simulink model "Quattrini_Michael_0001070264"  (R2023b)
settings: Solver=FixedStepAuto  StartTime=0.0  StopTime=1.2  FixedStep=5.0e-7  RelTol=1e-3
values from neighbouring files (symbols this model uses):
  carrier_period = 1/carrier_frequency    (= 2.5e-06)    [Quattrini_Michael_p0001070264.m]
  current_saturation = 9.2    [Quattrini_Michael_p0001070264.m]
  kfi = 1/317 * (60/(2*pi))    (= 0.0301239639922)    [Quattrini_Michael_p0001070264.m]
  ki_c = 3050    [Quattrini_Michael_p0001070264.m]
  ki_w = 0.0001    [Quattrini_Michael_p0001070264.m]
  kp_c = 18    [Quattrini_Michael_p0001070264.m]
  kp_w = 0.150    (= 0.15)    [Quattrini_Michael_p0001070264.m]
  load_torque_slope = 5.856e-5    (= 5.856e-05)    [Quattrini_Michael_p0001070264.m]
  nominal_speed = 6930*2*pi/60    (= 725.707902979)    [Quattrini_Michael_p0001070264.m]
  source_internal_resistance = 0.30    (= 0.3)    [Quattrini_Michael_p0001070264.m]
  supply_voltage = 30    [Quattrini_Michael_p0001070264.m]
  total_inertia = (rotor_inertia + load_inertia) * 10^(-7)    (= 3.38e-05)    [Quattrini_Michael_p0001070264.m]
  winding_resistance = 0.32    [Quattrini_Michael_p0001070264.m]
libraries: nesl_utility x12, ee_lib x10, fl_lib x8, simulink x3
settings Model: Creator=vince  LastModifiedBy=Utente
settings ModelReferenceCC: EnableRefExpFcnMdlSchedulingChecks=on

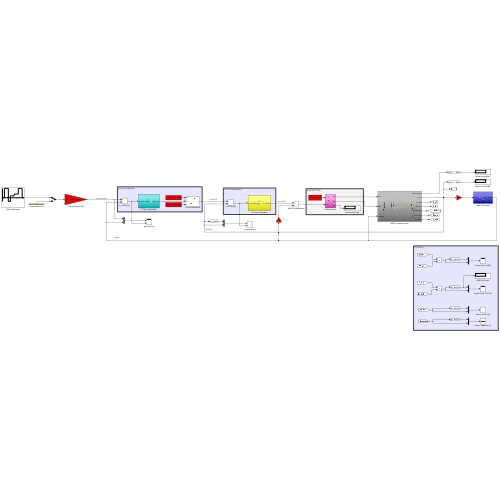
[thumbnail: Simulink's stored preview of the top-level diagram]
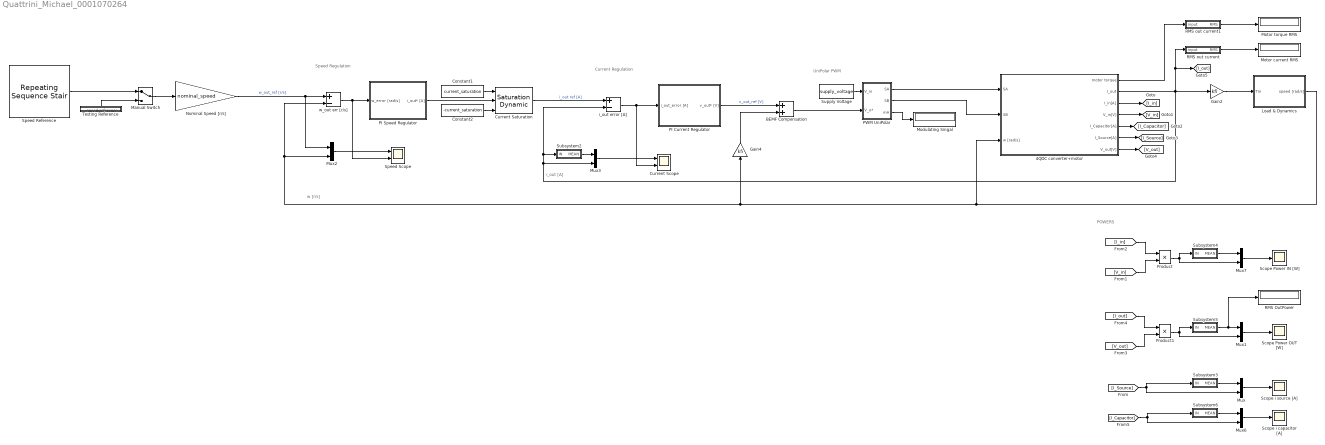
== system Quattrini_Michael_0001070264 ==
  note: w [r/s]
  note: i_out [A]
  note: Speed Regulation
  note: Current Regulation
  note: UniPolar PWM
  note: POWERS
  4QDC converter+motor : Subsystem
  BEMF Compensation : Sum
  Constant1 : Constant  Value=current_saturation
  Constant2 : Constant  Value=-current_saturation
  Current Saturation : simulink/Discontinuities/Saturation Dynamic  OutMin=[]  OutMax=[]  OutDataTypeStr=Inherit: Same as second input  OutDataType=fixdt(1, 16)  OutScaling=2^-10  DoSatur=off
  Current Scope : Scope  NumInputPorts=2
  Gain2 : Gain  Gain=kfi
  Gain4 : Gain  Gain=kfi
  Load & Dynamics : Subsystem
  Manual Switch : ManualSwitch
  Modulating Singal : Display
  Motor current RMS : Display
  Motor torque RMS : Display
  Mux{,1..3,6..7} (6 alike) : Mux  Inputs=2
  Nominal Speed [r/s] : Gain  Gain=nominal_speed
  PI Current Regulator : Subsystem
  PI Speed Regulator : Subsystem
  PWM UniPolar : Subsystem
  Product : Product
  Product1 : Product
  RMS OutPower : Display
  RMS out current : Subsystem  mask{t=1.2}
      mask prompts: t "Integrating time T [s]"
      mask DialogControl DescTextVar Prompt: Mean value calculator over period T
  RMS out current1 : Subsystem  mask{t=1.2}
      mask prompts: t "Integrating time T [s]"
      mask DialogControl DescTextVar Prompt: Mean value calculator over period T
  Scope Power IN [W] : Scope
  Scope Power OUT [W] : Scope
  Scope i capacitor [A] : Scope
  Scope i source [A] : Scope
  Speed Reference : simulink/Sources/Repeating Sequence Stair  OutValues=[0 1.25 1.25 -0.5 0.25 0.25 0.50 0.50 1.25 1.25 1/667^2]  tsamp=0.1  OutMin=[]  OutMax=[]  OutDataTypeStr=double  OutputDataTypeScalingMode=double  OutDataType=fixdt(0,8)  ConRadixGroup=Best Precision: Vector-wise  OutScaling=2^-12
  Speed Scope : Scope  NumInputPorts=2
  Subsystem2 : Subsystem  mask{carrierPeriod=carrier_period}
  Subsystem3 : Subsystem  mask{carrierPeriod=carrier_period}
  Subsystem4 : Subsystem  mask{carrierPeriod=carrier_period}
  Subsystem5 : Subsystem  mask{carrierPeriod=carrier_period}
  Subsystem6 : Subsystem  mask{carrierPeriod=carrier_period}
  Supply Voltage : Constant  Value=supply_voltage
  Testing Reference : Subsystem
      settings: PortSchema="{\"entries\":[{\"content\":{\"sides\":[{\"content\":{\"connectorIds\":[]},\"type\":\"ConnectorPlacement.EquallySpacedRectSide\",\"uuid\":\"1e7059c8-be33-4535-aff5-f50a3743a179\"},{\"content\":{\"connectorIds\":[],\"side\":\"RIGHT\"},\"type\":\"ConnectorPlacement.EquallySpacedRectSide\",\"uuid\":\"f13681df-83b1-4c0d-b4d9-acb75cd15713\"},{\"content\":{\"connectorIds\":[\"Out1\"],\"side\":\"TOP\"},\"type\":\"ConnectorPlacement.EquallySpacedRectSide\",\"uuid\":\"954c28a6-7a50-41b4-bd4f-7c1c0b7465e3\"}]},\"type\":\"ConnectorPlacement.EquallySpacedConnector\",\"uuid\":\"8215162a-5d8c-4681-a7f6-9e1221fb7294\"}],\"packageUris\":[\"http://schema.mathworks.com/mf0/Connector/R2020b\"],\"version\":\"1.0\"}"
  i_out error [A] : Sum  Inputs=+-
  w_out err [r/s] : Sum  Inputs=+-
  wires:
  BEMF Compensation/1 -> PWM UniPolar/2(V_o*)
  Current Saturation/1 -> i_out error [A]/1  "i_out ref [A]"
  i_out error [A]/1 -> PI Current Regulator/1(i_out_error [A]), Current Scope/2
  w_out err [r/s]/1 -> Speed Scope/2, PI Speed Regulator/1(w_error [rad/s])
  Nominal Speed [r/s]/1 -> w_out err [r/s]/1, Mux2/1  "w_out_ref [r/s]"
  Gain4/1 -> BEMF Compensation/2
  Subsystem2/1(MEAN) -> Mux3/1
  PI Speed Regulator/1(i_out* [A]) -> Current Saturation/2
  Constant1/1 -> Current Saturation/1
  Manual Switch/1 -> Nominal Speed [r/s]/1
  Speed Reference/1 -> Manual Switch/1
  Testing Reference/1(speed reference) -> Manual Switch/2
  Gain2/1 -> Load & Dynamics/1(Tm)
  Load & Dynamics/1(speed [rad/s]) -> Gain4/1, w_out err [r/s]/2, Mux2/2, 4QDC converter+motor/3(w [rad/s])
  Supply Voltage/1 -> PWM UniPolar/1(V_in)
  PWM UniPolar/3(mA) -> Modulating Singal/1
  PWM UniPolar/2(SB) -> 4QDC converter+motor/2(SB)
  PWM UniPolar/1(SA) -> 4QDC converter+motor/1(SA)
  Mux3/1 -> Current Scope/1
  Mux2/1 -> Speed Scope/1
  PI Current Regulator/1(v_out* [V]) -> BEMF Compensation/1  "v_out_ref [V]"
  4QDC converter+motor/2(I_out) -> Mux3/2, Subsystem2/1(IN), i_out error [A]/2, Gain2/1, RMS out current/1(input), [I_out]
  4QDC converter+motor/3(I_in[A]) -> [I_in]
  4QDC converter+motor/4(V_in[V]) -> [V_in]
  4QDC converter+motor/6(I_Source[A]) -> [I_Source]
  4QDC converter+motor/5(I_Capacitor[A]) -> [I_Capacitor]
  RMS out current1/1(RMS) -> Motor torque RMS/1
  RMS out current/1(RMS) -> Motor current RMS/1
  4QDC converter+motor/1(motor torque) -> RMS out current1/1(input)
  Product/1 -> Mux7/2, Subsystem4/1(IN)
  Subsystem4/1(MEAN) -> Mux7/1
  [V_out] -> Product1/2
  [V_in] -> Product/2
  [I_out] -> Product1/1
  Product1/1 -> Mux1/2, Subsystem5/1(IN)
  Mux1/1 -> Scope Power OUT [W]/1
  Subsystem5/1(MEAN) -> RMS OutPower/1, Mux1/1
  [I_in] -> Product/1
  Mux7/1 -> Scope Power IN [W]/1
  [I_Source] -> Subsystem3/1(IN), Mux/2
  Mux6/1 -> Scope i capacitor [A]/1
  Subsystem3/1(MEAN) -> Mux/1
  Mux/1 -> Scope i source [A]/1
  [I_Capacitor] -> Mux6/2, Subsystem6/1(IN)
  Subsystem6/1(MEAN) -> Mux6/1
  Constant2/1 -> Current Saturation/3
  4QDC converter+motor/7(V_out[V]) -> [V_out]

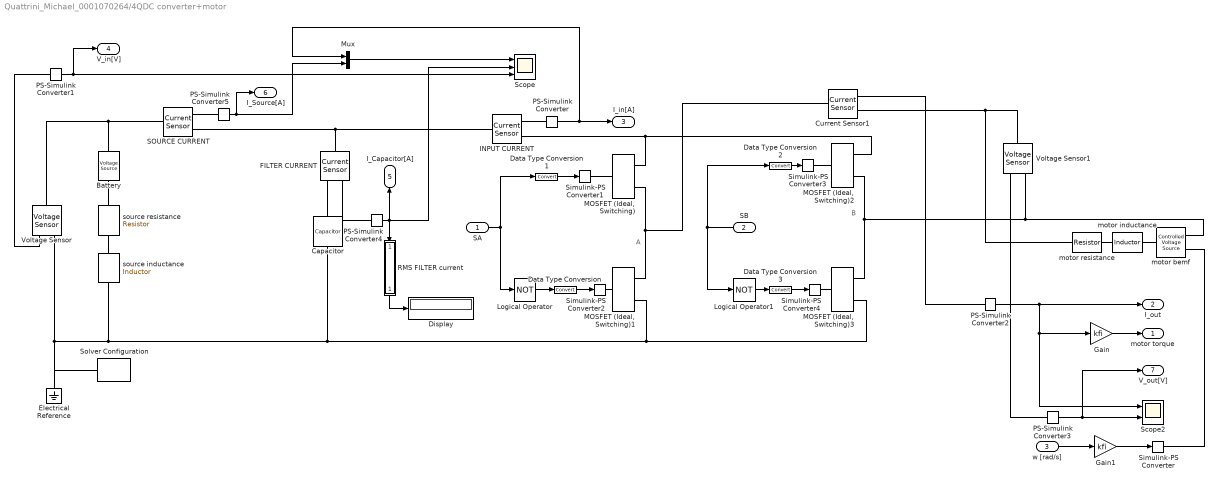
== system Quattrini_Michael_0001070264/4QDC converter+motor ==
  note: B
  note: A
  SA : Inport
  SB : Inport  Port=2
  w [rad/s] : Inport  Port=3
  Battery : ee_lib/Sources/Voltage Source  dc_voltage=supply_voltage V  ac_voltage=0 V  ac_shift=0 rad  ac_frequency=60 Hz  noise_mode=0  PSD=0 V^2/Hz  sample_time=1e-3 s  repeatability=1  user_seed=0  auto_seed=3890346746  i_specify=off  i_priority=None  i=0 A  i_nominal_specify=off  i_nominal_unit=A  i_nominal_value=1  v_specify=off  v_priority=None  v=0 V  v_nominal_specify=off  v_nominal_unit=V  v_nominal_value=1
  Capacitor : ee_lib/Passive/Capacitor  cap_option=ee.enum.passive.capacitor.capOption.const  c=filter_capacitance F  Cvec=[1e-05, 1e-06] F  Vvec=[0, 10] V  CV_table_symmetry=1  f_vec=[1, 10] kHz  DFext_vec=[.8, 1.2]  enable_C_tol=0  averaging_period=0 s  C_tol=5  tol_distribution=1  nSigma=4  r=0.001 Ohm  g=0 1/Ohm  enable_operating_limits=0  operating_limit_action=2  max_working_voltage_range=[-25, 25] V  power_rating=1 W  enable_faults=ee.enum.enable.no  fault_action=simscape.enum.assert.action.none  Cscale_faulted=100  R_faulted=1e-3 Ohm  G_faulted=0 1/Ohm  tau_fault=1e-3 s  fault_trigger=ee.enum.faults.faultTrigger.temporal  t_fault=1 s  max_permissible_voltage_range=[-100, 100] V  t_fail_on_voltage=1 s  i_specify=off  i_priority=None  i=0 A  i_nominal_specify=off  i_nominal_unit=A  i_nominal_value=1  v_specify=off  v_priority=None  v=0 V  v_nominal_specify=off  v_nominal_unit=V  v_nominal_value=1  vc_specify=off  vc_priority=High  vc=0 V  vc_nominal_specify=off  vc_nominal_unit=V  vc_nominal_value=1
  Current Sensor1 : fl_lib/Electrical/Electrical Sensors/Current Sensor
  Data Type Conversion{,1..3} (4 alike) : DataTypeConversion  SaturateOnIntegerOverflow=off  RndMeth=Floor
  Display : Display
  Electrical Reference : fl_lib/Electrical/Electrical Elements/Electrical Reference
  FILTER CURRENT : fl_lib/Electrical/Electrical Sensors/Current Sensor
  Gain : Gain  Gain=kfi
  Gain1 : Gain  Gain=kfi
  INPUT CURRENT : fl_lib/Electrical/Electrical Sensors/Current Sensor
  Logical Operator : Logic  Operator=NOT  AllPortsSameDT=off  OutDataTypeStr=boolean
  Logical Operator1 : Logic  Operator=NOT  AllPortsSameDT=off  OutDataTypeStr=boolean
  MOSFET (Ideal, Switching){,1..3} (4 alike) : ee_lib/Semiconductors & Converters/MOSFET (Ideal, Switching)  port_option=ee.enum.controlport.ps  Rds=0.01 Ohm  Goff=1e-6 1/Ohm  Vth=0.5 V  diode_param=1  diode_Vf=0.8 V  diode_Ron=0.001 Ohm  diode_Goff=1e-5 1/Ohm  diode_C=50e-9 F  diode_iRM=-235 A  diode_iF=300 A  diode_idot=-50 A/us  diode_trr_param=1  diode_trr_factor=3  diode_trr=15 us  diode_Qrr=1500 s*uA  ids_specify=off  ids_priority=None  ids=0 A  ids_nominal_specify=off  ids_nominal_unit=A  ids_nominal_value=1  vds_specify=off  vds_priority=None  vds=0 V  vds_nominal_specify=off  vds_nominal_unit=V  vds_nominal_value=1  vgs_specify=off  vgs_priority=None  vgs=0 V  vgs_nominal_specify=off  vgs_nominal_unit=V  vgs_nominal_value=1  thermal_loss_option=ee.enum.converters.thermalLossOption.constantvalues  Von_data=[0, 1.8, 3.2, 6, 10, 16; 0, 2, 5.5, 9.5, 15, 25] V  Tj=[298.15, 448.15] K  Iout_data=[0, 20, 40, 60, 80, 100] A  Eon_data=[0, 55.04, 124.57, 235.53, 362.12; 0, 71.25, 161.25, 304.88, 468.75] * 1e-6 J  Eoff_data=[0, 18, 30, 56.1, 76.5; 0, 22.5, 37.5, 70.13, 95.63] * 1e-6 J  Eon_data_3D=[zeros(2, 5, 3)] J  Eoff_data_3D=[zeros(2, 5, 3)] J  Tj_loss=[298.15, 448.15] K  Iout_data_loss=[0, 10, 20, 30, 40] A  tabulateWithVds=false  Vds_loss=[0, 150, 300] V  Eon_scalar=22.86e-3 J  Eoff_scalar=17.14e-3 J  Voff=300 V  Iout_scalar=600 A  useCurrentFromPreviousCycle=false  useVoltageFromPreviousCycle=false  diodeModelType=ee.enum.converters.diodeModelType.pwl  diodeTableType=ee.enum.diode.tableType.IfMat  diode_IfMat=[.07, .12, .19, 1.75, 4.24, 7.32, 11.2; .16, .3, .72, 2.14, 4.02, 6.35, 9.12] A  diode_VfMat=[.9, 1.15, 1.25, 1.5, 1.75, 2.17, 2.6, 2.85; .58, .68, .75, 1.1, 1.38, 1.77, 2.27, 2.7] V  diode_TjVec=[25, 125] degC  diode_VfVec=[.5, .7, .9, 1.3, 1.7, 2.1, 2.5] V  diode_IfVec=[.1, .2, .5, 1, 2, 4, 7, 10] A  diode_Vr=-600 V  diode_Ls=150 nH  diode_Erec=0.03 J  diode_rec_loss_model=ee.enum.diode.reverseRecoveryModel.fixed  diode_ErecVal=0 J  diode_scaleWithIandV=true  diode_ErecMat=zeros(2, 3) J  diode_TjrecVec=[298.15, 398.15] K  diode_IfrecVec=[.1, 1, 10] A  diode_IrecVal=10 A  diode_VrecVal=10 V  diode_tFilter=1 / 1000 / 100 s  thermal_network_parameterization=ee.enum.thermalNetworkTopology.external  Rth=[.03, .2] K/W  Rth_Cauer=[.03, .1, .2] K/W  Rth_Foster=[.03, .2] K/W  thermal_mass_parameterization=ee.enum.thermalNetwork.timeconstant  thermal_mass=[3, 25] J/K  thermal_mass_Cauer=[3, 10, 25] J/K  thermal_mass_Foster=[33, 50] J/K  thermal_time_constant=[.1, 5] s  thermal_time_constant_Cauer=[.1, 1, 5] s  thermal_time_constant_Foster=[1, 10] s  thermal_mass_initial_temperatures=[25, 25] degC  thermal_mass_initial_temperatures_Cauer=[25, 25, 25] degC  junction_thermal_mass=0.1 J/K  Tvec_initial_Foster=[25, 25, 25, 25] degC  no_thermal_network=0  junction_temperature_specify=off  junction_temperature_priority=None  junction_temperature=25 degC  junction_temperature_nominal_specify=off  junction_temperature_nominal_unit=degC  junction_temperature_nominal_value=1  Qj_specify=off  Qj_priority=None  Qj=0 W  Qj_nominal_specify=off  Qj_nominal_unit=W  Qj_nominal_value=1  accumulatedSwitchingLosses_specify=off  accumulatedSwitchingLosses_priority=None  accumulatedSwitchingLosses=0 J
  Mux : Mux  Inputs=2
  PS-Simulink Converter{,1..5} (6 alike) : nesl_utility/PS-Simulink Converter  PhysicalDomain=network_engine_domain  SubClassName=ps_output  LeftPortType=input  RightPortType=output  PseudoPeriodic=off  Frequencies=[]  VectorFormat=1-D array  Unit=inherit  AffineConversion=off
  RMS FILTER current : Subsystem  mask{t=1.2}
      mask prompts: t "Integrating time T [s]"
      mask DialogControl DescTextVar Prompt: Mean value calculator over period T
  SOURCE CURRENT : fl_lib/Electrical/Electrical Sensors/Current Sensor
  Scope : Scope  NumInputPorts=3
  Scope2 : Scope  NumInputPorts=2
  Simulink-PS Converter{,1..4} (5 alike) : nesl_utility/Simulink-PS Converter  PhysicalDomain=network_engine_domain  SubClassName=ps_input  LeftPortType=input  RightPortType=output  PseudoPeriodic=off  Frequencies=[]  NoiseDistribution=none  NoiseParameters=[]  Unit=1  AffineConversion=off  FilteringAndDerivatives=provide  SimscapeFilterOrder=1  InputFilterTimeConstant=0.001  UdotUserProvided=0
  Solver Configuration : nesl_utility/Solver Configuration  PhysicalDomain=network_engine_domain  SubClassName=solver  LeftPortType=input  RightPortType=generic  Tones=[]  Harmonics=[]  SimulateNoise=off  Profile=off  UseLocalSampling=off  EnableSwitchedLinearOptims=on  FrequencyDomain=off  UseCCode=off  RelTol=0.001  AbsTol=1e-06  MinStep=1e-09  ToWorkspace=off  RevertToSquareIcSolve=off  NumHomotopyIterations=100  PhasorMode=off  PhasorModeNumHarmonics=1  ConsistencySolver=NEWTON_FTOL  IndexReductionMethod=DerivativeReplacement  DoDC=off  ResidualTolerance=1e-09  ConsistencyTolSource=GLOBAL  ConsistencyAbsTol=0.001  ConsistencyRelTol=0.001  ConsistencyTolFactor=0.001  UseLocalSolver=off  LocalSolverChoice=NE_BACKWARD_EULER_ADVANCER  ResolveIndetEquations=on  FunctionEvalNumThread=1  LocalSolverSampleTime=0.001  DoFixedCost=off  MaxNonlinIter=3  MaxModeIter=2  ComputeImpulses=off  ImpulseIterations=2  LinearAlgebra=auto  LinearAlgebraNumThread=0  EquationFormulation=NE_TIME_EF  DelaysMemoryBudget=1024  AutomaticFiltering=on  FilteringTimeConstant=0.001  PartitionStorageMethod=AS_NEEDED  PartitionMemoryBudget=1024  PartitionMethod=ROBUST  MultibodyUseLocalSolver=off  MultibodyLocalSolverChoice=ODE1  MultibodyLocalSolverSampleTime=0.001
  Voltage Sensor : fl_lib/Electrical/Electrical Sensors/Voltage Sensor
  Voltage Sensor1 : fl_lib/Electrical/Electrical Sensors/Voltage Sensor
  motor inductance : ee_lib/Passive/Inductor  l=winding_inductance H  enable_L_tol=0  L_tol=20  tol_distribution=1  nSigma=4  r=0 Ohm  g=1e-9 1/Ohm  enable_operating_limits=0  operating_limit_action=2  max_working_current=1 A  power_rating=1 W  enable_faults=ee.enum.enable.no  fault_action=simscape.enum.assert.action.none  lambdaPercent=50  k_faulted=0.9999  turnsShort=0  openCct=0  groundShort=0  groundShortG=0 1/Ohm  tau_fault=1e-3 s  fault_trigger=ee.enum.faults.faultTrigger.temporal  t_fault=1 s  max_permissible_voltage=100 V  n_fail_on_voltage=1  max_permissible_current=1 A  t_fail_on_current=1 s  i_L_specify=off  i_L_priority=High  i_L=0 A  i_L_nominal_specify=off  i_L_nominal_unit=A  i_L_nominal_value=1
  "motor resistance " : ee_lib/Passive/Resistor  R=winding_resistance Ohm  enable_R_tol=0  R_tol=5  tol_distribution=1  nSigma=4  enable_operating_limits=0  operating_limit_action=2  power_rating=1 W  max_working_voltage=100 V  enable_faults=ee.enum.enable.no  fault_action=simscape.enum.assert.action.none  R_faulted=inf Ohm  fault_trigger=ee.enum.faults.faultTrigger.temporal  t_fault=1 s  max_permissible_current=1 A  t_fail_on_current=1 s  noise_mode=0  Tdevice=25 degC  sample_time=1e-3 s  repeatability=1  user_seed=0  auto_seed=545404223  faulted_specify=off  faulted_priority=None  faulted=0  power_derating_T1=70 degC  power_derating_T2=155 degC  operating_temperature_range_vec=[-50, 150] degC  alpha=3.93e-3 1/K  Tmeas=25 degC  thermal_mass=100 J/K  temperature_specify=off  temperature_priority=High  temperature=298.15 K  temperature_nominal_specify=off  temperature_nominal_unit=K  temperature_nominal_value=1
  motor bemf : fl_lib/Electrical/Electrical Sources/Controlled Voltage Source
  source inductance : ee_lib/Passive/Inductor  l=source_internal_inductance H  enable_L_tol=0  L_tol=20  tol_distribution=1  nSigma=4  r=0 Ohm  g=1e-9 1/Ohm  enable_operating_limits=0  operating_limit_action=2  max_working_current=1 A  power_rating=1 W  enable_faults=ee.enum.enable.no  fault_action=simscape.enum.assert.action.none  lambdaPercent=50  k_faulted=0.9999  turnsShort=0  openCct=0  groundShort=0  groundShortG=0 1/Ohm  tau_fault=1e-3 s  fault_trigger=ee.enum.faults.faultTrigger.temporal  t_fault=1 s  max_permissible_voltage=100 V  n_fail_on_voltage=1  max_permissible_current=1 A  t_fail_on_current=1 s  i_L_specify=off  i_L_priority=High  i_L=0 A  i_L_nominal_specify=off  i_L_nominal_unit=A  i_L_nominal_value=1
  source resistance : ee_lib/Passive/Resistor  R=source_internal_resistance Ohm  enable_R_tol=0  R_tol=5  tol_distribution=1  nSigma=4  enable_operating_limits=0  operating_limit_action=2  power_rating=1 W  max_working_voltage=100 V  enable_faults=ee.enum.enable.no  fault_action=simscape.enum.assert.action.none  R_faulted=inf Ohm  fault_trigger=ee.enum.faults.faultTrigger.temporal  t_fault=1 s  max_permissible_current=1 A  t_fail_on_current=1 s  noise_mode=0  Tdevice=25 degC  sample_time=1e-3 s  repeatability=1  user_seed=0  auto_seed=3922919431  faulted_specify=off  faulted_priority=None  faulted=0  power_derating_T1=70 degC  power_derating_T2=155 degC  operating_temperature_range_vec=[-50, 150] degC  alpha=3.93e-3 1/K  Tmeas=25 degC  thermal_mass=100 J/K  temperature_specify=off  temperature_priority=High  temperature=298.15 K  temperature_nominal_specify=off  temperature_nominal_unit=K  temperature_nominal_value=1
  motor torque : Outport
  I_out : Outport  Port=2
  I_in[A] : Outport  Port=3
  V_in[V] : Outport  Port=4
  I_Capacitor[A] : Outport  Port=5
  I_Source[A] : Outport  Port=6
  V_out[V] : Outport  Port=7
  wires:
  SB/1 -> Data Type Conversion2/1, Logical Operator1/1
  SA/1 -> Logical Operator/1, Data Type Conversion1/1
  PS-Simulink Converter2/1 -> Scope2/1, Gain/1, I_out/1
  Gain/1 -> motor torque/1
  w [rad/s]/1 -> Gain1/1
  Gain1/1 -> Simulink-PS Converter/1
  PS-Simulink Converter3/1 -> V_out[V]/1, Scope2/2
  Logical Operator/1 -> Data Type Conversion/1
  Data Type Conversion/1 -> Simulink-PS Converter2/1
  Data Type Conversion1/1 -> Simulink-PS Converter1/1
  Data Type Conversion2/1 -> Simulink-PS Converter3/1
  Logical Operator1/1 -> Data Type Conversion3/1
  Data Type Conversion3/1 -> Simulink-PS Converter4/1
  PS-Simulink Converter/1 -> Mux/1, I_in[A]/1
  Mux/1 -> Scope/1
  PS-Simulink Converter1/1 -> V_in[V]/1, Scope/3
  PS-Simulink Converter5/1 -> I_Source[A]/1, Mux/2
  PS-Simulink Converter4/1 -> I_Capacitor[A]/1, Scope/2, RMS FILTER current/1(input)
  RMS FILTER current/1(RMS) -> Display/1
  connections:
  Voltage Sensor/LConn1 -- Battery/LConn1 -- SOURCE CURRENT/LConn1
  "MOSFET (Ideal, Switching)1"/RConn2 -- Capacitor/RConn1 -- Voltage Sensor/RConn2 -- Electrical Reference/LConn1 -- Solver Configuration/RConn1 -- source inductance/RConn1 -- "MOSFET (Ideal, Switching)3"/RConn2
  "motor resistance "/RConn1 -- motor inductance/LConn1
  Simulink-PS Converter3/RConn1 -- "MOSFET (Ideal, Switching)2"/LConn1
  INPUT CURRENT/RConn2 -- "MOSFET (Ideal, Switching)"/RConn1 -- "MOSFET (Ideal, Switching)2"/RConn1
  motor bemf/RConn2 -- "MOSFET (Ideal, Switching)2"/RConn2 -- "MOSFET (Ideal, Switching)3"/RConn1 -- Voltage Sensor1/RConn2
  INPUT CURRENT/RConn1 -- PS-Simulink Converter/LConn1
  Voltage Sensor/RConn1 -- PS-Simulink Converter1/LConn1
  Simulink-PS Converter1/RConn1 -- "MOSFET (Ideal, Switching)"/LConn1
  Simulink-PS Converter/RConn1 -- motor bemf/RConn1
  "MOSFET (Ideal, Switching)"/RConn2 -- Current Sensor1/LConn1 -- "MOSFET (Ideal, Switching)1"/RConn1
  Simulink-PS Converter4/RConn1 -- "MOSFET (Ideal, Switching)3"/LConn1
  Simulink-PS Converter2/RConn1 -- "MOSFET (Ideal, Switching)1"/LConn1
  motor inductance/RConn1 -- motor bemf/LConn1
  Current Sensor1/RConn2 -- Voltage Sensor1/LConn1 -- "motor resistance "/LConn1
  Current Sensor1/RConn1 -- PS-Simulink Converter2/LConn1
  Voltage Sensor1/RConn1 -- PS-Simulink Converter3/LConn1
  source inductance/LConn1 -- source resistance/RConn1
  source resistance/LConn1 -- Battery/RConn1
  SOURCE CURRENT/RConn2 -- FILTER CURRENT/LConn1 -- INPUT CURRENT/LConn1
  FILTER CURRENT/RConn2 -- Capacitor/LConn1
  FILTER CURRENT/RConn1 -- PS-Simulink Converter4/LConn1
  SOURCE CURRENT/RConn1 -- PS-Simulink Converter5/LConn1

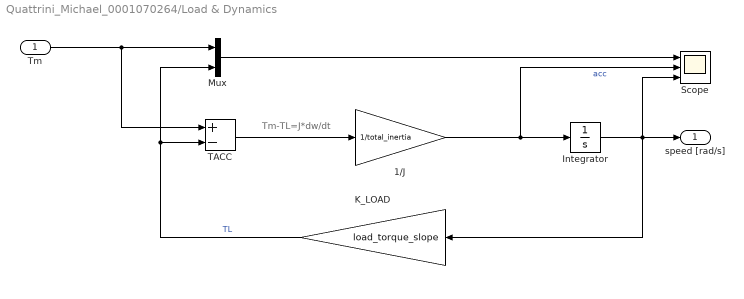
== system Quattrini_Michael_0001070264/Load & Dynamics ==
  note: Tm-TL=J*dw/dt
  Tm : Inport
  1/J : Gain  Gain=1/total_inertia
  Integrator : Integrator
  K_LOAD : Gain  Gain=load_torque_slope
  Mux : Mux  Inputs=2
  Scope : Scope  NumInputPorts=3
  TACC : Sum  Inputs=+-
  speed [rad/s] : Outport
  wires:
  Tm/1 -> Mux/1, TACC/1
  1/J/1 -> Scope/2, Integrator/1  "acc"
  K_LOAD/1 -> Mux/2, TACC/2  "TL"
  Integrator/1 -> K_LOAD/1, Scope/3, speed [rad/s]/1
  TACC/1 -> 1/J/1
  Mux/1 -> Scope/1

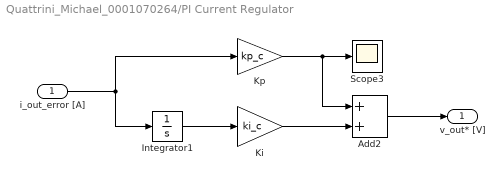
== system Quattrini_Michael_0001070264/PI Current Regulator ==
  i_out_error [A] : Inport
  Add2 : Sum
  Integrator1 : Integrator
  Ki : Gain  Gain=ki_c
  Kp : Gain  Gain=kp_c
  Scope3 : Scope
  v_out* [V] : Outport
  wires:
  Add2/1 -> v_out* [V]/1
  Kp/1 -> Add2/1, Scope3/1
  Ki/1 -> Add2/2
  Integrator1/1 -> Ki/1
  i_out_error [A]/1 -> Kp/1, Integrator1/1

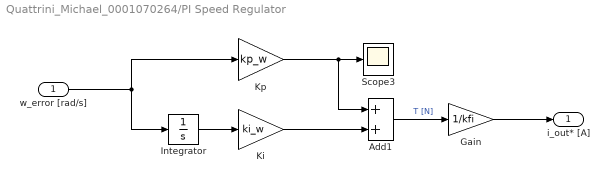
== system Quattrini_Michael_0001070264/PI Speed Regulator ==
  w_error [rad/s] : Inport
  Add1 : Sum
  Gain : Gain  Gain=1/kfi
  Integrator : Integrator
  Ki : Gain  Gain=ki_w
  Kp : Gain  Gain=kp_w
  Scope3 : Scope
  i_out* [A] : Outport
  wires:
  w_error [rad/s]/1 -> Integrator/1, Kp/1
  Kp/1 -> Add1/1, Scope3/1
  Integrator/1 -> Ki/1
  Ki/1 -> Add1/2
  Add1/1 -> Gain/1  "T [N]"
  Gain/1 -> i_out* [A]/1

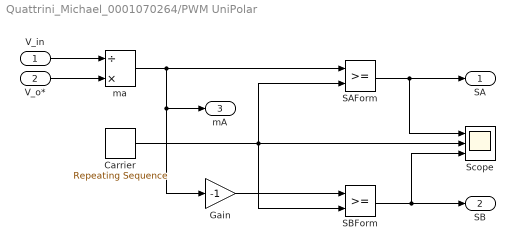
== system Quattrini_Michael_0001070264/PWM UniPolar ==
  V_in : Inport
  V_o* : Inport  Port=2
  Carrier : simulink/Sources/Repeating Sequence  rep_seq_t=[0 carrier_period/2 carrier_period]  rep_seq_y=[-1 1 -1]
  Gain : Gain  Gain=-1
  SAForm : RelationalOperator  OutDataTypeStr=boolean  RndMeth=Simplest  InputSameDT=off
  SBForm : RelationalOperator  OutDataTypeStr=boolean  RndMeth=Simplest  InputSameDT=off
  Scope : Scope  NumInputPorts=3
  ma : Product  Inputs=/*
  SA : Outport
  SB : Outport  Port=2
  mA : Outport  Port=3
  wires:
  Carrier/1 -> SBForm/2, SAForm/2, Scope/2
  Gain/1 -> SBForm/1
  SBForm/1 -> SB/1, Scope/3
  SAForm/1 -> Scope/1, SA/1
  V_in/1 -> ma/1
  V_o*/1 -> ma/2
  ma/1 -> mA/1, Gain/1, SAForm/1

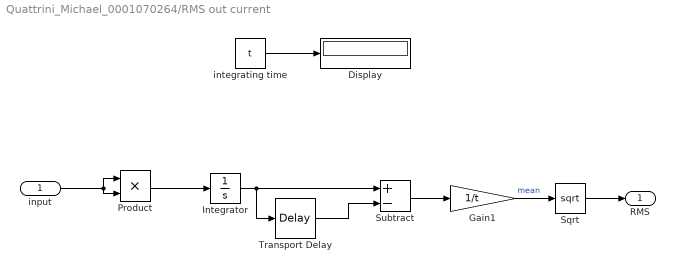
== system Quattrini_Michael_0001070264/RMS out current ==
  input : Inport
  Display : Display
  Gain1 : Gain  Gain=1/t
  Integrator : Integrator
  Product : Product
  Sqrt : Sqrt
  Subtract : Sum  Inputs=+-
  Transport Delay : TransportDelay  DelayTime=t
  integrating time : Constant  Value=t
  RMS : Outport
  wires:
  integrating time/1 -> Display/1
  Transport Delay/1 -> Subtract/2
  Integrator/1 -> Transport Delay/1, Subtract/1
  Subtract/1 -> Gain1/1
  input/1 -> Product/1, Product/2
  Product/1 -> Integrator/1
  Sqrt/1 -> RMS/1
  Gain1/1 -> Sqrt/1  "mean"

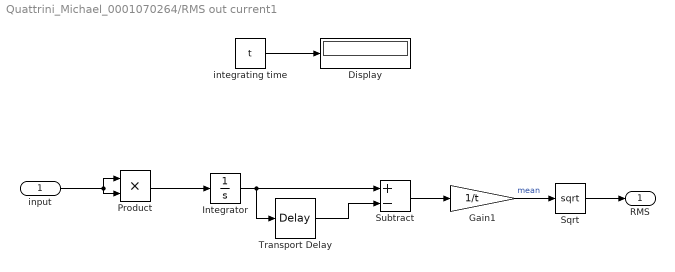
== system Quattrini_Michael_0001070264/RMS out current1 ==
  input : Inport
  Display : Display
  Gain1 : Gain  Gain=1/t
  Integrator : Integrator
  Product : Product
  Sqrt : Sqrt
  Subtract : Sum  Inputs=+-
  Transport Delay : TransportDelay  DelayTime=t
  integrating time : Constant  Value=t
  RMS : Outport
  wires:
  integrating time/1 -> Display/1
  Transport Delay/1 -> Subtract/2
  Integrator/1 -> Transport Delay/1, Subtract/1
  Subtract/1 -> Gain1/1
  input/1 -> Product/1, Product/2
  Product/1 -> Integrator/1
  Sqrt/1 -> RMS/1
  Gain1/1 -> Sqrt/1  "mean"

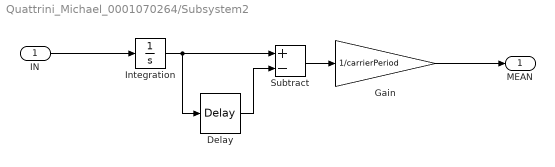
== system Quattrini_Michael_0001070264/Subsystem2 ==
  IN : Inport
  Delay : TransportDelay  DelayTime=carrierPeriod
  Gain : Gain  Gain=1/carrierPeriod
  Integration : Integrator
  Subtract : Sum  Inputs=+-
  MEAN : Outport
  wires:
  Delay/1 -> Subtract/2
  Integration/1 -> Delay/1, Subtract/1
  Subtract/1 -> Gain/1
  IN/1 -> Integration/1
  Gain/1 -> MEAN/1

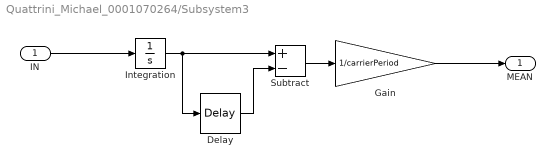
== system Quattrini_Michael_0001070264/Subsystem3 ==
  IN : Inport
  Delay : TransportDelay  DelayTime=carrierPeriod
  Gain : Gain  Gain=1/carrierPeriod
  Integration : Integrator
  Subtract : Sum  Inputs=+-
  MEAN : Outport
  wires:
  Delay/1 -> Subtract/2
  Integration/1 -> Delay/1, Subtract/1
  Subtract/1 -> Gain/1
  IN/1 -> Integration/1
  Gain/1 -> MEAN/1

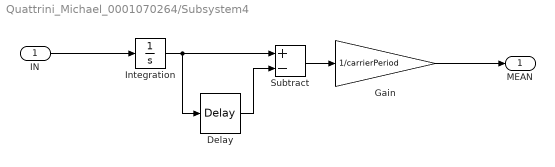
== system Quattrini_Michael_0001070264/Subsystem4 ==
  IN : Inport
  Delay : TransportDelay  DelayTime=carrierPeriod
  Gain : Gain  Gain=1/carrierPeriod
  Integration : Integrator
  Subtract : Sum  Inputs=+-
  MEAN : Outport
  wires:
  Delay/1 -> Subtract/2
  Integration/1 -> Delay/1, Subtract/1
  Subtract/1 -> Gain/1
  IN/1 -> Integration/1
  Gain/1 -> MEAN/1

== system Quattrini_Michael_0001070264/Subsystem5 ==
  IN : Inport
  Delay : TransportDelay  DelayTime=carrierPeriod
  Gain : Gain  Gain=1/carrierPeriod
  Integration : Integrator
  Subtract : Sum  Inputs=+-
  MEAN : Outport
  wires:
  Delay/1 -> Subtract/2
  Integration/1 -> Delay/1, Subtract/1
  Subtract/1 -> Gain/1
  IN/1 -> Integration/1
  Gain/1 -> MEAN/1

== system Quattrini_Michael_0001070264/Subsystem6 ==
  IN : Inport
  Delay : TransportDelay  DelayTime=carrierPeriod
  Gain : Gain  Gain=1/carrierPeriod
  Integration : Integrator
  Subtract : Sum  Inputs=+-
  MEAN : Outport
  wires:
  Delay/1 -> Subtract/2
  Integration/1 -> Delay/1, Subtract/1
  Subtract/1 -> Gain/1
  IN/1 -> Integration/1
  Gain/1 -> MEAN/1

== system Quattrini_Michael_0001070264/Testing Reference ==
  0 to 100% Step at 10ms : Step  Time=10 * 10^(-3)  SampleTime=0
  "0 to 25% Step at 210ms " : Step  Time=210 * 10^(-3)  After=0.25  SampleTime=0
  Sum : Sum
  speed reference : Outport
  wires:
  "0 to 25% Step at 210ms "/1 -> Sum/2
  0 to 100% Step at 10ms/1 -> Sum/1
  Sum/1 -> speed reference/1

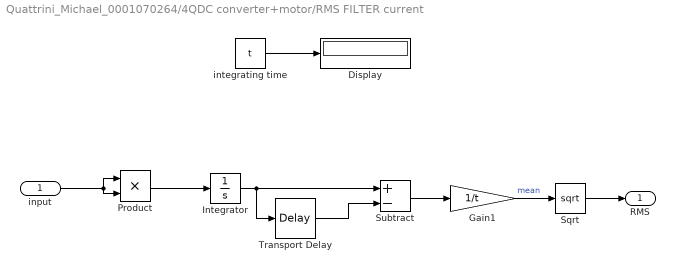
== system Quattrini_Michael_0001070264/4QDC converter+motor/RMS FILTER current ==
  input : Inport
  Display : Display
  Gain1 : Gain  Gain=1/t
  Integrator : Integrator
  Product : Product
  Sqrt : Sqrt
  Subtract : Sum  Inputs=+-
  Transport Delay : TransportDelay  DelayTime=t
  integrating time : Constant  Value=t
  RMS : Outport
  wires:
  integrating time/1 -> Display/1
  Transport Delay/1 -> Subtract/2
  Integrator/1 -> Transport Delay/1, Subtract/1
  Subtract/1 -> Gain1/1
  input/1 -> Product/1, Product/2
  Product/1 -> Integrator/1
  Sqrt/1 -> RMS/1
  Gain1/1 -> Sqrt/1  "mean"
